simulink model "baseline_auto_parcel_loading_process"  (R2026a)
settings: Solver=VariableStepAuto  StopTime=500  MaxStep=0.05
libraries: sim3dlib x36
(part 2 of 5)

== matlab function baseline_auto_parcel_loading_process/BoxSizeFunction ==
  data: box_type output; box_length output; box_width output; box_height output; load_done input; package_count output
function [box_type, box_length, box_width, box_height, package_count] = BoxSizeFunction(load_done)
% BoxSizeFunction
% 연속 상차용 랜덤 택배 크기 생성 함수
%
% load_done이 0 -> 1로 바뀌는 순간,
% 다음 상차 사이클에서 사용할 새 택배 종류를 랜덤 생성한다.
%
% 출력 단위:
% box_length, box_width, box_height = m

persistent selected_type
persistent count
persistent prev_load_done

if isempty(selected_type)
    selected_type = randi(4);
    count = 1;
    prev_load_done = 0;
end

% load_done 상승 에지 감지
rising_edge = (prev_load_done == 0) && (load_done == 1);

% 상차 완료 순간 다음 택배 생성
if rising_edge
    selected_type = randi(4);
    count = count + 1;
end

prev_load_done = load_done;

box_type = selected_type;
package_count = count;

% 우체국 택배 1~4호 예시 치수
% 실제 제작 박스 치수에 맞춰 나중에 수정 가능
% [length, width, height], 단위: m
if box_type == 1
    real_length = 0.220;
    real_width  = 0.190;
    real_height = 0.090;
elseif box_type == 2
    real_length = 0.270;
    real_width  = 0.180;
    real_height = 0.150;
elseif box_type == 3
    real_length = 0.340;
    real_width  = 0.250;
    real_height = 0.210;
else
    real_length = 0.410;
    real_width  = 0.310;
    real_height = 0.280;
end

% 2:1 축소 스케일
scale = 0.5;

box_length = real_length * scale;
box_width  = real_width  * scale;
box_height = real_height * scale;

== stateflow chart baseline_auto_parcel_loading_process/MainController ==
  state LOAD_FINISHED
    entry:
    lift_cmd = 0;
    target_z = 0.0;
    state_id = 14;
    door_cmd = 0;
    platform_fold_cmd = 0;
    rotator_cmd = 0;
    pusher_cmd = 0;
    % 핵심: 상차 phase 종료이므로 스토퍼 올림
    stopper_cmd = 0;
    floor1_conv_cmd = 0;
    floor2_conv_cmd = 0;
    floor3_conv_cmd = 0;
    load_done = 0;
    spawn_pkg = 0;
  state NO_STORAGE
    entry:
    lift_cmd = 0;
    target_z = 0.0;
    state_id = 13;
    door_cmd = 1;
    platform_fold_cmd = 1;
    rotator_cmd = 0;
    pusher_cmd = 0;
    stopper_cmd = 0;
    floor1_conv_cmd = 0;
    floor2_conv_cmd = 0;
    floor3_conv_cmd = 0;
    load_done = 0;
    spawn_pkg = 0;
  state ROTATOR_RETURN_HOME
    entry:
    lift_cmd = 0;
    target_z = 0.0;
    state_id = 15;
    door_cmd = 1;
    platform_fold_cmd = 1;
    rotator_cmd = 2;
    pusher_cmd = 0;
    stopper_cmd = 0;
    floor1_conv_cmd = 0;
    floor2_conv_cmd = 0;
    floor3_conv_cmd = 0;
    load_done = 0;
    spawn_pkg = 0;
  state COMPLETE
    entry:
    lift_cmd = 0;
    target_z = 0.0;
    state_id = 12;
    door_cmd = 1;
    platform_fold_cmd = 1;
    rotator_cmd = 0;
    pusher_cmd = 0;
    stopper_cmd = 0;
    floor1_conv_cmd = 0;
    floor2_conv_cmd = 0;
    floor3_conv_cmd = 0;
    load_done = 0;
    spawn_pkg = 0;
  state IDLE
    entry:
    lift_cmd = 0;
    target_z = 0.0;
    state_id = 0;
    door_cmd = 1;
    platform_fold_cmd = 1;
    rotator_cmd = 0;
    pusher_cmd = 0;
    stopper_cmd = 0;
    floor1_conv_cmd = 0;
    floor2_conv_cmd = 0;
    floor3_conv_cmd = 0;
    load_done = 0;
    spawn_pkg = 0;
  state SELECT_TARGET_FLOOR
    entry:
    lift_cmd = 0;
    if target_floor == 1
    target_z = 0.0;
    elseif target_floor == 2
    target_z = 0.27;
    elseif target_floor == 3
    target_z = 0.54;
    else
    target_z = 0.0;
    end
    state_id = 4;
    door_cmd = 1;
    platform_fold_cmd = 1;
    rotator_cmd = 0;
    pusher_cmd = 0;
    stopper_cmd = 0;
    floor1_conv_cmd = 0;
    floor2_conv_cmd = 0;
    floor3_conv_cmd = 0;
    load_done = 0;
    spawn_pkg = 0;
  state WAIT_PACKAGE
    entry:
    lift_cmd = 0;
    target_z = 0.0;
    state_id = 2;
    door_cmd = 1;
    platform_fold_cmd = 1;
    rotator_cmd = 0;
    pusher_cmd = 0;
    stopper_cmd = 0;
    floor1_conv_cmd = 0;
    floor2_conv_cmd = 0;
    floor3_conv_cmd = 0;
    load_done = 0;
    spawn_pkg = 1;
  state SCAN_AND_ROTATE
    entry:
    lift_cmd = 0;
    target_z = 0.0;
    state_id = 3;
    door_cmd = 1;
    platform_fold_cmd = 1;
    rotator_cmd = 1;
    pusher_cmd = 0;
    stopper_cmd = 0;
    floor1_conv_cmd = 0;
    floor2_conv_cmd = 0;
    floor3_conv_cmd = 0;
    load_done = 0;
    spawn_pkg = 0;
  state MOVE_TO_TARGET_FLOOR
    during:
    if target_floor == 1
    target_z = 0.0;
    elseif target_floor == 2
    target_z = 0.27;
    elseif target_floor == 3
    target_z = 0.54;
    else
    target_z = 0.0;
    end
    if platform_z < target_z - 0.0001
    lift_cmd = 1;
    else
    lift_cmd = 0;
    end
    state_id = 5;
    door_cmd = 1;
    platform_fold_cmd = 1;
    rotator_cmd = 0;
    pusher_cmd = 0;
    stopper_cmd = 0;
    floor1_conv_cmd = 0;
    floor2_conv_cmd = 0;
    floor3_conv_cmd = 0;
    load_done = 0;
    spawn_pkg = 0;
  state PLATFORM_UNFOLD
    entry:
    lift_cmd = 0;
    target_z = 0.0;
    state_id = 1;
    door_cmd = 1;
    platform_fold_cmd = 1;
    rotator_cmd = 0;
    pusher_cmd = 0;
    stopper_cmd = 0;
    floor1_conv_cmd = 0;
    floor2_conv_cmd = 0;
    floor3_conv_cmd = 0;
    load_done = 0;
    spawn_pkg = 0;
  state LOAD_REGISTER
    entry:
    lift_cmd = 0;
    if target_floor == 1
    target_z = 0.0;
    floor1_conv_cmd = 0;
    floor2_conv_cmd = 0;
    floor3_conv_cmd = 0;
    elseif target_floor == 2
    target_z = 0.27;
    floor1_conv_cmd = 0;
    floor2_conv_cmd = 0;
    floor3_conv_cmd = 0;
    elseif target_floor == 3
    target_z = 0.54;
    floor1_conv_cmd = 0;
    floor2_conv_cmd = 0;
    floor3_conv_cmd = 0;
    else
    target_z = 0.0;
    floor1_conv_cmd = 0;
    floor2_conv_cmd = 0;
    floor3_conv_cmd = 0;
    end
    state_id = 17;
    door_cmd = 1;
    platform_fold_cmd = 1;
    rotator_cmd = 0;
    pusher_cmd = 0;
    % 핵심: 아직 상차 phase 중이므로 스토퍼는 계속 내려둔다
    stopper_cmd = 1;
    % 여기서 상차 완료 신호 발생
    load_done = 1;
    spawn_pkg = 0;
  state PUSH_TO_BELT4
    entry:
    lift_cmd = 0;
    if target_floor == 1
    target_z = 0.0;
    floor1_conv_cmd = 1;
    floor2_conv_cmd = 0;
    floor3_conv_cmd = 0;
    elseif target_floor == 2
    target_z = 0.27;
    floor1_conv_cmd = 0;
    floor2_conv_cmd = 1;
    floor3_conv_cmd = 0;
    elseif target_floor == 3
    target_z = 0.54;
    floor1_conv_cmd = 0;
    floor2_conv_cmd = 0;
    floor3_conv_cmd = 1;
    else
    target_z = 0.0;
    floor1_conv_cmd = 0;
    floor2_conv_cmd = 0;
    floor3_conv_cmd = 0;
    end
    state_id = 7;
    door_cmd = 1;
    platform_fold_cmd = 1;
    rotator_cmd = 0;
    pusher_cmd = 1;
    stopper_cmd = 1;
    load_done = 0;
    spawn_pkg = 0;
  state PACKING
    entry:
    lift_cmd = 0;
    if target_floor == 1
    target_z = 0.0;
    floor1_conv_cmd = 1;
    floor2_conv_cmd = 0;
    floor3_conv_cmd = 0;
    elseif target_floor == 2
    target_z = 0.27;
    floor1_conv_cmd = 0;
    floor2_conv_cmd = 1;
    floor3_conv_cmd = 0;
    elseif target_floor == 3
    target_z = 0.54;
    floor1_conv_cmd = 0;
    floor2_conv_cmd = 0;
    floor3_conv_cmd = 1;
    else
    target_z = 0.0;
    floor1_conv_cmd = 1;
    floor2_conv_cmd = 0;
    floor3_conv_cmd = 0;
    end
    state_id = 8;
    door_cmd = 1;
    platform_fold_cmd = 1;
    rotator_cmd = 0;
    pusher_cmd = 0;
    stopper_cmd = 1;
    load_done = 0;
    spawn_pkg = 0;
  state PUSHER_RETURN_HOME
    entry:
    lift_cmd = 0;
    if target_floor == 1
    target_z = 0.0;
    floor1_conv_cmd = 1;
    floor2_conv_cmd = 0;
    floor3_conv_cmd = 0;
    elseif target_floor == 2
    target_z = 0.27;
    floor1_conv_cmd = 0;
    floor2_conv_cmd = 1;
    floor3_conv_cmd = 0;
    elseif target_floor == 3
    target_z = 0.54;
    floor1_conv_cmd = 0;
    floor2_conv_cmd = 0;
    floor3_conv_cmd = 1;
    else
    target_z = 0.0;
    floor1_conv_cmd = 0;
    floor2_conv_cmd = 0;
    floor3_conv_cmd = 0;
    end
    state_id = 16;
    door_cmd = 1;
    platform_fold_cmd = 1;
    rotator_cmd = 0;
    pusher_cmd = 2;
    stopper_cmd = 1;
    load_done = 0;
    spawn_pkg = 0;
  state MOVE_DOWN
    entry:
    target_z = 0.0;
    lift_cmd = -1;
    state_id = 10;
    door_cmd = 1;
    platform_fold_cmd = 1;
    rotator_cmd = 0;
    pusher_cmd = 0;
    stopper_cmd = 1;
    floor1_conv_cmd = 0;
    floor2_conv_cmd = 0;
    floor3_conv_cmd = 0;
    spawn_pkg = 0;
  state PLATFORM_FOLD
    entry:
    lift_cmd = 0;
    target_z = 0.0;
    state_id = 11;
    door_cmd = 1;
    platform_fold_cmd = 0;
    rotator_cmd = 0;
    pusher_cmd = 0;
    stopper_cmd = 0;
    floor1_conv_cmd = 0;
    floor2_conv_cmd = 0;
    floor3_conv_cmd = 0;
    spawn_pkg = 0;
  state STOPPER_DOWN
    entry:
    lift_cmd = 0;
    if target_floor == 1
    target_z = 0.0;
    elseif target_floor == 2
    target_z = 0.27;
    elseif target_floor == 3
    target_z = 0.54;
    else
    target_z = 0.0;
    end
    state_id = 6;
    door_cmd = 1;
    platform_fold_cmd = 1;
    rotator_cmd = 0;
    pusher_cmd = 0;
    stopper_cmd = 1;
    floor1_conv_cmd = 0;
    floor2_conv_cmd = 0;
    floor3_conv_cmd = 0;
    load_done = 0;
    spawn_pkg = 0;
  IDLE -> LOAD_FINISHED [order 2] : [after(1, sec) && loading_enable == 0]
  COMPLETE -> LOAD_FINISHED [order 2] : [after(1, sec) && loading_enable == 0]
  SELECT_TARGET_FLOOR -> NO_STORAGE [order 2] : [storage_available == 0]
  (default) -> IDLE
  IDLE -> PLATFORM_UNFOLD [order 1] : [after(1, sec) && loading_enable == 1]
  SELECT_TARGET_FLOOR -> MOVE_TO_TARGET_FLOOR [order 1] : [storage_available == 1]
  COMPLETE -> IDLE [order 1] : [after(1, sec) && loading_enable == 1]
  SCAN_AND_ROTATE -> ROTATOR_RETURN_HOME : [rotation_done == 1]
  ROTATOR_RETURN_HOME -> SELECT_TARGET_FLOOR : [rotator_home_done == 1]
  PLATFORM_UNFOLD -> WAIT_PACKAGE : [after(1, sec)]
  WAIT_PACKAGE -> SCAN_AND_ROTATE : [after(1, sec)]
  PLATFORM_FOLD -> COMPLETE : [after(1, sec)]
  MOVE_TO_TARGET_FLOOR -> STOPPER_DOWN : [platform_z >= target_z - 0.0001]
  MOVE_DOWN -> PLATFORM_FOLD : [platform_z <= 0.0001]
  LOAD_REGISTER -> MOVE_DOWN : [after(0.1, sec)]
  STOPPER_DOWN -> PUSH_TO_BELT4 : [stopper_down_done == 1]
  PACKING -> LOAD_REGISTER : [moving_arrive_done == 1]
  PUSHER_RETURN_HOME -> PACKING : [pusher_home_done == 1]
  PUSH_TO_BELT4 -> PUSHER_RETURN_HOME : [push_done == 1]
  data: target_floor input; platform_z input; lift_cmd output; target_z output; state_id output; door_cmd output; platform_fold_cmd output; rotator_cmd output; pusher_cmd output; stopper_cmd output; floor1_conv_cmd output; floor2_conv_cmd output; floor3_conv_cmd output; load_done output; storage_available input; loading_enable input; rotation_done input; rotator_home_done input; push_done input; pusher_home_done input; stopper_down_done input; spawn_pkg output; moving_arrive_done input

== matlab function baseline_auto_parcel_loading_process/BoxRotationFunction ==
  data: box_length input; box_insert_length output; box_width input; desired_box_yaw output; box_yaw input; rotator_target_angle output
function [box_insert_length, desired_box_yaw, rotator_target_angle] = BoxRotationFunction(box_length, box_width, box_yaw)
% BoxRotationFunction
% 랜덤하게 놓인 택배 yaw를 기준으로,
% 컨베이어 진행방향 점유 길이가 최소가 되도록 필요한 회전각을 계산한다.
%
% 입력:
%   box_length : 택배 긴 방향 길이 [m]
%   box_width  : 택배 짧은 방향 길이 [m]
%   box_yaw    : 카메라/YOLO가 인식한 현재 택배 yaw [deg]
%
% 출력:
%   box_insert_length     : 회전 후 컨베이어 진행방향으로 차지하는 길이 [m]
%   desired_box_yaw       : 목표 택배 yaw [deg]
%   rotator_target_angle  : 회전판이 회전해야 하는 보정각 [deg]

% 적재 효율을 위해 짧은 변이 진행방향을 향하도록 한다.
% 여기서는 단순히:
% - box_length <= box_width이면 현재 0 deg 방향이 유리
% - box_length > box_width이면 90 deg 방향이 유리
%
% 실제로는 카메라 좌표계와 컨베이어 진행방향 정의에 따라
% desired_box_yaw 기준을 조정해야 한다.

if box_length <= box_width
    box_insert_length = box_length;
    desired_box_yaw = 0;
else
    box_insert_length = box_width;
    desired_box_yaw = 90;
end

% 현재 yaw에서 목표 yaw까지 필요한 회전각
raw_angle = desired_box_yaw - box_yaw;

% 회전각을 -90 ~ 90 deg 범위로 정규화
rotator_target_angle = normalizeToMinus90To90(raw_angle);


function angle_out = normalizeToMinus90To90(angle_in)
% angle_in을 -90 ~ 90 범위로 정규화

angle_out = angle_in;

while angle_out > 90
    angle_out = angle_out - 180;
end

while angle_out < -90
    angle_out = angle_out + 180;
end

== matlab function baseline_auto_parcel_loading_process/FloorStorageUpdate ==
  data: load_done input; floor1_used_length output; target_floor input; box_insert_length input; floor2_used_length output; floor3_used_length output; floor1_count output; floor2_count output; floor3_count output; package_id input; floor1_queue output; floor2_queue output; floor3_queue output; unload_done input; target_package_id input; target_unload_floor input; target_package_length output
function [floor1_used_length, floor2_used_length, floor3_used_length, floor1_count, floor2_count, floor3_count, floor1_queue, floor2_queue, floor3_queue, target_package_length] = FloorStorageUpdate(load_done, target_floor, box_insert_length, package_id, unload_done, target_package_id, target_unload_floor)
% FloorStorageUpdate
% 상차 완료 시:
%   1) 선택된 층 used_length 증가
%   2) 선택된 층 count 증가
%   3) 선택된 층 queue 뒤에 package_id 저장
%   4) package_id별 box_insert_length 저장
%
% 하차 완료 시:
%   1) 대상 층 queue에서 target_package_id 삭제
%   2) 대상 층 count 감소
%   3) target_package_id에 저장된 길이만큼 used_length 감소
%
% queue는 column vector [QUEUE_MAX x 1] 형태로 통일한다.

persistent f1_used f2_used f3_used
persistent f1_count f2_count f3_count
persistent q1 q2 q3
persistent package_lengths
persistent prev_load_done prev_unload_done

QUEUE_MAX = 50;
PACKAGE_MAX = 1000;

if isempty(f1_used)
    % 초기 적재 길이
    f1_used = 0.40;
    f2_used = 0.45;
    f3_used = 0.20;

    % 이번 시뮬레이션에서 새로 상차된 택배 개수
    f1_count = 0;
    f2_count = 0;
    f3_count = 0;

    % 층별 큐: column vector로 통일
    q1 = zeros(QUEUE_MAX, 1);
    q2 = zeros(QUEUE_MAX, 1);
    q3 = zeros(QUEUE_MAX, 1);

    % package_id별 택배 진행방향 길이 저장
    package_lengths = zeros(PACKAGE_MAX, 1);

    prev_load_done = 0;
    prev_unload_done = 0;
end

% 상승 에지 감지
load_rising_edge = (prev_load_done == 0) && (load_done == 1);
unload_rising_edge = (prev_unload_done == 0) && (unload_done == 1);

% 현재 target_package_id의 저장된 길이 조회
target_idx = int32(target_package_id);
target_package_length = 0;

if target_idx >= 1 && target_idx <= PACKAGE_MAX
    target_package_length = package_lengths(target_idx);
end

% =========================
% 상차 업데이트
% =========================
if load_rising_edge
    pkg_idx = int32(package_id);

    % package_id별 길이 저장
    if pkg_idx >= 1 && pkg_idx <= PACKAGE_MAX
        package_lengths(pkg_idx) = box_insert_length;
    end

    if target_floor == 1
        if f1_count < QUEUE_MAX
            f1_count = f1_count + 1;
            q1(f1_count) = package_id;
            f1_used = f1_used + box_insert_length;
        end

    elseif target_floor == 2
        if f2_count < QUEUE_MAX
            f2_count = f2_count + 1;
            q2(f2_count) = package_id;
            f2_used = f2_used + box_insert_length;
        end

    elseif target_floor == 3
        if f3_count < QUEUE_MAX
            f3_count = f3_count + 1;
            q3(f3_count) = package_id;
            f3_used = f3_used + box_insert_length;
        end
    end
end

% =========================
% 하차 업데이트
% =========================
if unload_rising_edge
    target_idx_for_unload = int32(target_package_id);
    removed_length = 0;

    if target_idx_for_unload >= 1 && target_idx_for_unload <= PACKAGE_MAX
        removed_length = package_lengths(target_idx_for_unload);
    end

    % 혹시 길이가 저장되어 있지 않으면 안전하게 현재 box_insert_length 사용
    if removed_length <= 0
        removed_length = box_insert_length;
    end

    if target_unload_floor == 1
        [q1, f1_count, removed] = removePackageFromQueue(q1, f1_count, target_package_id, QUEUE_MAX);

        if removed == 1
            f1_used = f1_used - removed_length;

            if f1_used < 0
                f1_used = 0;
            end

            if target_idx_for_unload >= 1 && target_idx_for_unload <= PACKAGE_MAX
                package_lengths(target_idx_for_unload) = 0;
            end
        end

    elseif target_unload_floor == 2
        [q2, f2_count, removed] = removePackageFromQueue(q2, f2_count, target_package_id, QUEUE_MAX);

        if removed == 1
            f2_used = f2_used - removed_length;

            if f2_used < 0
                f2_used = 0;
            end

            if target_idx_for_unload >= 1 && target_idx_for_unload <= PACKAGE_MAX
                package_lengths(target_idx_for_unload) = 0;
            end
        end

    elseif target_unload_floor == 3
        [q3, f3_count, removed] = removePackageFromQueue(q3, f3_count, target_package_id, QUEUE_MAX);

        if removed == 1
            f3_used = f3_used - removed_length;

            if f3_used < 0
                f3_used = 0;
            end

            if target_idx_for_unload >= 1 && target_idx_for_unload <= PACKAGE_MAX
                package_lengths(target_idx_for_unload) = 0;
            end
        end
    end
end

prev_load_done = load_done;
prev_unload_done = unload_done;

% 하차 업데이트 이후 target_package_length 다시 계산
target_idx = int32(target_package_id);
target_package_length = 0;

if target_idx >= 1 && target_idx <= PACKAGE_MAX
    target_package_length = package_lengths(target_idx);
end

floor1_used_length = f1_used;
floor2_used_length = f2_used;
floor3_used_length = f3_used;

floor1_count = f1_count;
floor2_count = f2_count;
floor3_count = f3_count;

floor1_queue = q1;
floor2_queue = q2;
floor3_queue = q3;


function [q_out, count_out, removed] = removePackageFromQueue(q_in, count_in, target_id, queue_max)
% q_in에서 target_id를 찾아 삭제하고, 뒤쪽 원소들을 앞으로 당긴다.

q_out = q_in;
count_out = count_in;
removed = 0;

remove_idx = 0;

for i = 1:queue_max
    if q_out(i) == target_id
        remove_idx = i;
        removed = 1;
        break;
    end
end

if removed == 1
    % 삭제 위치부터 한 칸씩 앞으로 당김
    for i = remove_idx:(queue_max - 1)
        q_out(i) = q_out(i + 1);
    end

    % 마지막 칸 비우기
    q_out(queue_max) = 0;

    % count 감소
    if count_out > 0
        count_out = count_out - 1;
    end
end

== matlab function baseline_auto_parcel_loading_process/TargetPackageFinder ==
  data: target_package_id input; target_found output; floor1_queue input; floor2_queue input; floor3_queue input; target_unload_floor output; target_package_index output
function [target_found, target_unload_floor, target_package_index] = TargetPackageFinder(target_package_id, floor1_queue, floor2_queue, floor3_queue)
% TargetPackageFinder
% target_package_id가 각 층 queue 중 어디에 있는지 찾는다.
%
% target_found:
%   0 = 못 찾음
%   1 = 찾음
%
% target_unload_floor:
%   0 = 못 찾음
%   1 = 1층
%   2 = 2층
%   3 = 3층
%
% target_package_index:
%   해당 층 queue 안에서 몇 번째인지
%   예: floor2_queue = [1 2 4 0 ...]에서 target_package_id=4이면 index=3

target_found = 0;
target_unload_floor = 0;
target_package_index = 0;

QUEUE_MAX = 50;

% 1층 검색
for i = 1:QUEUE_MAX
    if floor1_queue(i) == target_package_id
        target_found = 1;
        target_unload_floor = 1;
        target_package_index = i;
        return;
    end
end

% 2층 검색
for i = 1:QUEUE_MAX
    if floor2_queue(i) == target_package_id
        target_found = 1;
        target_unload_floor = 2;
        target_package_index = i;
        return;
    end
end

% 3층 검색
for i = 1:QUEUE_MAX
    if floor3_queue(i) == target_package_id
        target_found = 1;
        target_unload_floor = 3;
        target_package_index = i;
        return;
    end
end

== matlab function baseline_auto_parcel_loading_process/UnloadPrepositionFunction ==
  data: unload_request input; preposition_active output; vehicle_stopped input; target_found input; target_unload_floor input; target_package_index input; sensor_count output; target_package_on_belt4 output; unload_floor1_conv_cmd output; unload_floor2_conv_cmd output; unload_floor3_conv_cmd output
function [preposition_active, sensor_count, target_package_on_belt4, unload_floor1_conv_cmd, unload_floor2_conv_cmd, unload_floor3_conv_cmd] = UnloadPrepositionFunction(unload_request, vehicle_stopped, target_found, target_unload_floor, target_package_index)
% UnloadPrepositionFunction
%
% 배송 중 하차 준비 단계 모델
%
% 목적:
% - 상차 완료 후 unload_request가 1이 되면 하차 준비 가능 상태가 된다.
% - 차량이 정차 중(vehicle_stopped == 1)일 때만 대상 층 컨베이어를 순환시킨다.
% - 모든 택배는 순서를 유지한 채 함께 순환한다고 가정한다.
% - target_package_index 위치의 택배가 slot 1, 즉 Belt4 상단/플랫폼 앞 하차공간에 오면
%   target_package_on_belt4 = 1 로 만든다.
%
% 핵심:
% - target_package_index = 1이면 이미 하차공간에 있는 것으로 판단한다.
% - target_package_index = 4이면 3칸 순환하면 하차공간에 온다.
%
% 출력:
% preposition_active       : 하차 준비 순환 중이면 1
% sensor_count             : 현재까지 순환된 칸 수
% target_package_on_belt4  : 대상 택배가 하차공간에 준비되면 1
% unload_floorN_conv_cmd   : 대상 층 순환 컨베이어 구동 명령

persistent count
persistent active
persistent done
persistent step_counter
persistent prev_unload_request
persistent last_target_floor
persistent last_target_index

% 몇 계산 step마다 택배 1개가 센서/하차공간 기준으로 이동했다고 볼지
% 값이 작을수록 순환 준비가 빠르게 보임
COUNT_INTERVAL = 20;

if isempty(count)
    count = 0;
    active = 0;
    done = 0;
    step_counter = 0;
    prev_unload_request = 0;
    last_target_floor = 0;
    last_target_index = 0;
end

% 기본 출력
preposition_active = active;
sensor_count = count;
target_package_on_belt4 = done;

unload_floor1_conv_cmd = 0;
unload_floor2_conv_cmd = 0;
unload_floor3_conv_cmd = 0;

% 하차 요청 상승 에지 감지
request_rising = (prev_unload_request == 0) && (unload_request == 1);

% 대상이 바뀌었는지도 확인
target_changed = (target_unload_floor ~= last_target_floor) || ...
                 (target_package_index ~= last_target_index);

% 새 하차 요청이 들어오거나 대상이 바뀌면 초기화
if request_rising || target_changed
    count = 0;
    active = 0;
    done = 0;
    step_counter = 0;

    last_target_floor = target_unload_floor;
    last_target_index = target_package_index;
end

prev_unload_request = unload_request;

% 유효하지 않은 조건이면 정지
if unload_request < 0.5 || target_found < 0.5 || target_unload_floor < 1 || target_unload_floor > 3 || target_package_index < 1
    active = 0;
    done = 0;
    count = 0;
    step_counter = 0;

    preposition_active = active;
    sensor_count = count;
    target_package_on_belt4 = done;
    return;
end

% target_package_index가 1이면 이미 Belt4 상단/플랫폼 앞 하차공간에 있다고 본다.
required_shift = target_package_index - 1;

if required_shift < 0
    required_shift = 0;
end

% 이미 필요한 만큼 순환했으면 준비 완료
if count >= required_shift
    active = 0;
    done = 1;

    unload_floor1_conv_cmd = 0;
    unload_floor2_conv_cmd = 0;
    unload_floor3_conv_cmd = 0;

    preposition_active = active;
    sensor_count = count;
    target_package_on_belt4 = done;
    return;
end

% 아직 준비가 안 끝났고, 차량이 정차 중이면 순환 시작/유지
if vehicle_stopped > 0.5
    active = 1;
else
    % 배송 중이지만 정차 상태가 아니면 현재 위치에서 멈춤
    active = 0;
end

% 하차 준비 동작
if active == 1 && done == 0

    % 대상 층 컨베이어만 순환
    if target_unload_floor == 1
        unload_floor1_conv_cmd = 1;
        unload_floor2_conv_cmd = 0;
        unload_floor3_conv_cmd = 0;

    elseif target_unload_floor == 2
        unload_floor1_conv_cmd = 0;
        unload_floor2_conv_cmd = 1;
        unload_floor3_conv_cmd = 0;

    elseif target_unload_floor == 3
        unload_floor1_conv_cmd = 0;
        unload_floor2_conv_cmd = 0;
        unload_floor3_conv_cmd = 1;
    end

    % 가상 센서/순환 카운트
    step_counter = step_counter + 1;

    if step_counter >= COUNT_INTERVAL
        step_counter = 0;
        count = count + 1;
    end

    % 필요한 순환 수에 도달하면 준비 완료
    if count >= required_shift
        done = 1;
        active = 0;

        unload_floor1_conv_cmd = 0;
        unload_floor2_conv_cmd = 0;
        unload_floor3_conv_cmd = 0;
    end
end

preposition_active = active;
sensor_count = count;
target_package_on_belt4 = done;

end

== stateflow chart baseline_auto_parcel_loading_process/UnloadController ==
  state U_IDLE
    during:
    unload_state_id = 0;
    belt4_reverse_cmd = 0;
    belt4_restore_cmd = 0;
    package_on_platform_from_floor = 0;
    unload_done = 0;
    % 기본 목표는 1층 복귀
    unload_target_z = 0.00;
    % 배송 중 하차 준비 단계에서는 실제 하차 전이므로
    % 플랫폼을 항상 1층으로 복귀시킨다.
    if delivery_arrived < 0.5
    if platform_z > 0.005
    unload_lift_cmd = -1;
    elseif platform_z < -0.005
    unload_lift_cmd = 1;
    else
    unload_lift_cmd = 0;
    end
    else
    % 배달 장소 도착 후에는 다음 하차 상태 전이를 기다림
    unload_lift_cmd = 0;
    end
  state U_WAIT_READY
    entry:
    unload_lift_cmd = 0;
    unload_target_z = 0.0;
    unload_state_id = 1;
    belt4_reverse_cmd = 0;
    belt4_restore_cmd = 0;
    package_on_platform_from_floor = 0;
    unload_done = 0;
  state U_MOVE_TO_TARGET_FLOOR
    during:
    unload_state_id = 2;
    belt4_reverse_cmd = 0;
    belt4_restore_cmd = 0;
    package_on_platform_from_floor = 0;
    unload_done = 0;
    if target_unload_floor == 1
    unload_target_z = 0.00;
    elseif target_unload_floor == 2
    unload_target_z = 0.27;
    elseif target_unload_floor == 3
    unload_target_z = 0.54;
    else
    unload_target_z = 0.00;
    end
    if platform_z < unload_target_z - 0.005
    unload_lift_cmd = 1;
    elseif platform_z > unload_target_z + 0.005
    unload_lift_cmd = -1;
    else
    unload_lift_cmd = 0;
    end
  state U_REVERSE_BELT4
    entry:
    unload_lift_cmd = 0;
    if target_unload_floor == 1
    unload_target_z = 0.0;
    elseif target_unload_floor == 2
    unload_target_z = 0.27;
    elseif target_unload_floor == 3
    unload_target_z = 0.54;
    else
    unload_target_z = 0.0;
    end
    unload_state_id = 3;
    belt4_reverse_cmd = 1;
    belt4_restore_cmd = 0;
    package_on_platform_from_floor = 0;
    unload_done = 0;
  state U_PACKAGE_ON_PLATFORM
    entry:
    unload_lift_cmd = 0;
    if target_unload_floor == 1
    unload_target_z = 0.0;
    elseif target_unload_floor == 2
    unload_target_z = 0.27;
    elseif target_unload_floor == 3
    unload_target_z = 0.54;
    else
    unload_target_z = 0.0;
    end
    unload_state_id = 4;
    belt4_reverse_cmd = 0;
    belt4_restore_cmd = 0;
    package_on_platform_from_floor = 1;
    unload_done = 0;
  state U_COMPLETE
    entry:
    unload_lift_cmd = 0;
    unload_target_z = 0.0;
    unload_state_id = 7;
    belt4_reverse_cmd = 0;
    belt4_restore_cmd = 0;
    package_on_platform_from_floor = 1;
    unload_done = 1;
  state U_RESTORE_BELT4
    entry:
    unload_lift_cmd = 0;
    if target_unload_floor == 1
    unload_target_z = 0.0;
    elseif target_unload_floor == 2
    unload_target_z = 0.27;
    elseif target_unload_floor == 3
    unload_target_z = 0.54;
    else
    unload_target_z = 0.0;
    end
    unload_state_id = 5;
    belt4_reverse_cmd = 0;
    belt4_restore_cmd = 1;
    package_on_platform_from_floor = 1;
    unload_done = 0;
  state U_MOVE_DOWN
    during:
    unload_target_z = 0.0;
    if platform_z > 0.0001
    unload_lift_cmd = -1;
    else
    unload_lift_cmd = 0;
    end
    unload_state_id = 6;
    belt4_reverse_cmd = 0;
    belt4_restore_cmd = 0;
    package_on_platform_from_floor = 1;
    unload_done = 0;
  (default) -> U_IDLE
  U_WAIT_READY -> U_MOVE_TO_TARGET_FLOOR : [delivery_arrived == 1]
  U_MOVE_TO_TARGET_FLOOR -> U_REVERSE_BELT4 : [(target_unload_floor == 1 && platform_z >= -0.005 && platform_z <= 0.005) || ...
      |  (target_unload_floor == 2 && platform_z >= 0.265 && platform_z <= 0.275) || ...
      |  (target_unload_floor == 3 && platform_z >= 0.535 && platform_z <= 0.545)]
  U_REVERSE_BELT4 -> U_PACKAGE_ON_PLATFORM : [after(1.5, sec)]
  U_IDLE -> U_WAIT_READY : [delivery_arrived > 0.5 && platform_deployed > 0.5 && target_package_on_belt4 > 0.5]
  U_COMPLETE -> U_IDLE : [after(0.1, sec)]
  U_PACKAGE_ON_PLATFORM -> U_RESTORE_BELT4 : [after(0.5, sec)]
  U_MOVE_DOWN -> U_COMPLETE : [platform_z <= 0.0001]
  U_RESTORE_BELT4 -> U_MOVE_DOWN : [after(1.5, sec)]
  data: target_package_on_belt4 input; target_unload_floor input; platform_z input; delivery_arrived input; unload_lift_cmd output; unload_target_z output; unload_state_id output; belt4_reverse_cmd output; belt4_restore_cmd output; package_on_platform_from_floor output; unload_done output; platform_deployed input

== matlab function baseline_auto_parcel_loading_process/MissionModeFunction ==
  data: floor1_count input; loading_enable output; floor2_count input; floor3_count input; load_target_count input; unload_request_auto output; total_loaded_count output; unload_done input; mission_phase output
function [loading_enable, unload_request_auto, total_loaded_count, mission_phase] = MissionModeFunction(floor1_count, floor2_count, floor3_count, load_target_count, unload_done)
% MissionModeFunction
%
% mission_phase:
% 0 = 상차 단계
% 1 = 하차 준비/하차 단계
% 2 = 전체 미션 완료

persistent phase
persistent prev_unload_done

if isempty(phase)
    phase = 0;
    prev_unload_done = 0;
end

total_loaded_count = floor1_count + floor2_count + floor3_count;

unload_rising_edge = (prev_unload_done == 0) && (unload_done == 1);

% 상차 완료 → 하차 단계
if phase == 0
    if total_loaded_count >= load_target_count
        phase = 1;
    end
end

% 모든 하차 대상 완료 → 미션 완료
if phase == 1
    if unload_rising_edge
        phase = 2;
    end
end

prev_unload_done = unload_done;

if phase == 0
    loading_enable = 1;
    unload_request_auto = 0;

elseif phase == 1
    loading_enable = 0;
    unload_request_auto = 1;

else
    loading_enable = 0;
    unload_request_auto = 0;
end

mission_phase = phase;

end

== matlab function baseline_auto_parcel_loading_process/CommandMuxFunction ==
  data: mission_phase input; final_lift_cmd output; load_lift_cmd input; load_target_z input; load_floor1_conv_cmd input; load_floor2_conv_cmd input; load_floor3_conv_cmd input; pre_floor1_conv_cmd input; pre_floor2_conv_cmd input; pre_floor3_conv_cmd input; unload_lift_cmd input; unload_target_z input; target_unload_floor input; belt4_reverse_cmd input; belt4_restore_cmd input; final_target_z output; final_floor1_conv_cmd output; final_floor2_conv_cmd output; final_floor3_conv_cmd output; final_floor1_belt4_cmd output; final_floor2_belt4_cmd output; final_floor3_belt4_cmd output
function [final_lift_cmd, final_target_z, ...
          final_floor1_conv_cmd, final_floor2_conv_cmd, final_floor3_conv_cmd, ...
          final_floor1_belt4_cmd, final_floor2_belt4_cmd, final_floor3_belt4_cmd] = ...
          CommandMuxFunction(mission_phase, ...
          load_lift_cmd, load_target_z, load_floor1_conv_cmd, load_floor2_conv_cmd, load_floor3_conv_cmd, ...
          pre_floor1_conv_cmd, pre_floor2_conv_cmd, pre_floor3_conv_cmd, ...
          unload_lift_cmd, unload_target_z, target_unload_floor, belt4_reverse_cmd, belt4_restore_cmd)
% CommandMuxFunction
% mission_phase에 따라 상차/하차 명령을 최종 장치 명령으로 선택한다.
%
% mission_phase:
%   0 = 상차 단계
%   1 = 하차 단계
%   2 = 미션 완료
%
% final_floorN_conv_cmd:
%   1 = 해당 층 전체 순환 컨베이어 시계방향 회전
%   0 = 정지
%
% final_floorN_belt4_cmd:
%  -1 = 4번 벨트 역회전, 택배를 플랫폼으로 하차
%   0 = 정지
%   1 = 4번 벨트 정방향 복귀

% 기본값: 전체 정지
final_lift_cmd = 0;
final_target_z = 0.0;

final_floor1_conv_cmd = 0;
final_floor2_conv_cmd = 0;
final_floor3_conv_cmd = 0;

final_floor1_belt4_cmd = 0;
final_floor2_belt4_cmd = 0;
final_floor3_belt4_cmd = 0;

% =========================
% 상차 단계
% =========================
if mission_phase == 0
    final_lift_cmd = load_lift_cmd;
    final_target_z = load_target_z;

    final_floor1_conv_cmd = load_floor1_conv_cmd;
    final_floor2_conv_cmd = load_floor2_conv_cmd;
    final_floor3_conv_cmd = load_floor3_conv_cmd;

    % 상차 중에는 벨트4 단독 역회전/복귀 명령 없음
    final_floor1_belt4_cmd = 0;
    final_floor2_belt4_cmd = 0;
    final_floor3_belt4_cmd = 0;

% =========================
% 하차 단계
% =========================
elseif mission_phase == 1
    final_lift_cmd = unload_lift_cmd;
    final_target_z = unload_target_z;

    % 하차 준비용 전체 순환 컨베이어 명령
    final_floor1_conv_cmd = pre_floor1_conv_cmd;
    final_floor2_conv_cmd = pre_floor2_conv_cmd;
    final_floor3_conv_cmd = pre_floor3_conv_cmd;
    
    % 4번 벨트 단독 동작 중에는 전체 순환 컨베이어 정지
    if belt4_reverse_cmd == 1 || belt4_restore_cmd == 1
        final_floor1_conv_cmd = 0;
        final_floor2_conv_cmd = 0;
        final_floor3_conv_cmd = 0;
    end

    % 하차 순간 4번 벨트 단독 명령
    if target_unload_floor == 1
        if belt4_reverse_cmd == 1
            final_floor1_belt4_cmd = -1;
        elseif belt4_restore_cmd == 1
            final_floor1_belt4_cmd = 1;
        else
            final_floor1_belt4_cmd = 0;
        end

    elseif target_unload_floor == 2
        if belt4_reverse_cmd == 1
            final_floor2_belt4_cmd = -1;
        elseif belt4_restore_cmd == 1
            final_floor2_belt4_cmd = 1;
        else
            final_floor2_belt4_cmd = 0;
        end

    elseif target_unload_floor == 3
        if belt4_reverse_cmd == 1
            final_floor3_belt4_cmd = -1;
        elseif belt4_restore_cmd == 1
            final_floor3_belt4_cmd = 1;
        else
            final_floor3_belt4_cmd = 0;
        end
    end

% =========================
% 미션 완료 또는 예외
% =========================
else
    final_lift_cmd = 0;
    final_target_z = 0;
    final_pusher_cmd = 0;

    final_floor1_conv_cmd = 0;
    final_floor2_conv_cmd = 0;
    final_floor3_conv_cmd = 0;

    final_belt4_reverse_cmd = 0;
    final_belt4_restore_cmd = 0;
end

== matlab function baseline_auto_parcel_loading_process/BoxPoseFunction ==
  data: load_done input; box_yaw output
function box_yaw = BoxPoseFunction(load_done)
% BoxPoseFunction
% 택배가 플랫폼 위에 랜덤하게 놓였다고 가정하고,
% 카메라/YOLO가 인식한 초기 yaw 각도를 생성한다.
%
% box_yaw 단위: deg
% 범위: -90 deg ~ 90 deg
%
% load_done이 0 -> 1로 바뀌면 다음 택배의 yaw를 새로 생성한다.

persistent current_yaw
persistent prev_load_done

if isempty(current_yaw)
    current_yaw = -90 + 180 * rand;
    prev_load_done = 0;
end

rising_edge = (prev_load_done == 0) && (load_done == 1);

if rising_edge
    current_yaw = -90 + 180 * rand;
end

prev_load_done = load_done;

box_yaw = current_yaw;

== matlab function baseline_auto_parcel_loading_process/RotatorControlFunction ==
  data: rotator_cmd input; rotator_vel output; rotator_target_angle input; rotator_angle input; rotation_done output; rotator_home_done output
function [rotator_vel, rotation_done, rotator_home_done] = RotatorControlFunction(rotator_cmd, rotator_target_angle, rotator_angle)
% RotatorControlFunction
% rotator_cmd에 따라 회전판을 제어한다.
%
% rotator_cmd:
%   0 = 정지
%   1 = 택배 yaw 보정 목표각(rotator_target_angle)으로 회전
%   2 = 회전판 원점 0 deg로 복귀
%
% rotation_done:
%   rotator_cmd == 1일 때 목표 보정각 도달 여부
%
% rotator_home_done:
%   rotator_cmd == 2일 때 0도 복귀 완료 여부

rotator_speed = 60;   % deg/s
angle_tol = 5.0;      % deg

rotator_vel = 0;
rotation_done = 0;
rotator_home_done = 0;

if rotator_cmd == 1
    target_angle = rotator_target_angle;
    error = target_angle - rotator_angle;

    if abs(error) <= angle_tol
        rotator_vel = 0;
        rotation_done = 1;
        rotator_home_done = 0;
    else
        if error > 0
            rotator_vel = rotator_speed;
        else
            rotator_vel = -rotator_speed;
        end
        rotation_done = 0;
        rotator_home_done = 0;
    end

elseif rotator_cmd == 2
    target_angle = 0;
    error = target_angle - rotator_angle;

    if abs(error) <= angle_tol
        rotator_vel = 0;
        rotation_done = 0;
        rotator_home_done = 1;
    else
        if error > 0
            rotator_vel = rotator_speed;
        else
            rotator_vel = -rotator_speed;
        end
        rotation_done = 0;
        rotator_home_done = 0;
    end

else
    rotator_vel = 0;
    rotation_done = 0;
    rotator_home_done = 0;
end

== matlab function baseline_auto_parcel_loading_process/PusherControlFunction ==
  data: pusher_cmd input; pusher_vel output; pusher_pos input; push_done output; pusher_home_done output; push_count output
function [pusher_vel, push_done, pusher_home_done, push_count] = PusherControlFunction(pusher_cmd, pusher_pos)
% PusherControlFunction
% pusher_cmd:
%   0 = 정지
%   1 = 전진, 택배를 벨트4 방향으로 밀기
%   2 = 원점 복귀

persistent count
persistent prev_push_done

if isempty(count)
    count = 0;
    prev_push_done = 0;
end

pusher_speed = 0.05;     % m/s
push_target_pos = 0.24;  % m
pos_tol = 0.002;         % m

pusher_vel = 0;
push_done = 0;
pusher_home_done = 0;

if pusher_cmd == 1
    if pusher_pos >= push_target_pos - pos_tol
        pusher_vel = 0;
        push_done = 1;
        pusher_home_done = 0;
    else
        pusher_vel = pusher_speed;
        push_done = 0;
        pusher_home_done = 0;
    end

elseif pusher_cmd == 2
    if pusher_pos <= pos_tol
        pusher_vel = 0;
        push_done = 0;
        pusher_home_done = 1;
    else
        pusher_vel = -pusher_speed;
        push_done = 0;
        pusher_home_done = 0;
    end

else
    pusher_vel = 0;
    push_done = 0;
    pusher_home_done = 0;
end

% push_done 상승 에지 카운트
if prev_push_done == 0 && push_done == 1
    count = count + 1;
end

prev_push_done = push_done;

push_count = count;

== matlab function baseline_auto_parcel_loading_process/StopperControlFunction ==
  data: stopper_cmd input; stopper_vel output; stopper_pos input; stopper_down_done output; stopper_up_done output
function [stopper_vel, stopper_down_done, stopper_up_done] = StopperControlFunction(stopper_cmd, stopper_pos)
% StopperControlFunction
% 스토퍼 위치 모델
%
% stopper_cmd:
%   0 = 스토퍼 올림
%   1 = 스토퍼 내림
%
% stopper_pos:
%   0 = 완전히 올라간 상태
%   1 = 완전히 내려간 상태
%
% stopper_vel:
%   스토퍼 위치 변화 속도 [1/s]
%
% stopper_down_done:
%   스토퍼가 완전히 내려갔는지
%
% stopper_up_done:
%   스토퍼가 완전히 올라갔는지

stopper_speed = 2.0;   % 1/s, 0에서 1까지 약 0.5초
pos_tol = 0.01;

stopper_vel = 0;
stopper_down_done = 0;
stopper_up_done = 0;

if stopper_cmd == 1
    % 스토퍼 내림
    if stopper_pos >= 1.0 - pos_tol
        stopper_vel = 0;
        stopper_down_done = 1;
        stopper_up_done = 0;
    else
        stopper_vel = stopper_speed;
        stopper_down_done = 0;
        stopper_up_done = 0;
    end

else
    % 스토퍼 올림
    if stopper_pos <= pos_tol
        stopper_vel = 0;
        stopper_down_done = 0;
        stopper_up_done = 1;
    else
        stopper_vel = -stopper_speed;
        stopper_down_done = 0;
        stopper_up_done = 0;
    end
end

== matlab function baseline_auto_parcel_loading_process/StopperCommandFunction ==
  data: mission_phase input; stopper_cmd_final output; loading_enable input
function stopper_cmd_final = StopperCommandFunction(mission_phase, loading_enable)
% StopperCommandFunction
% 스토퍼는 택배 1개마다 올렸다 내리는 것이 아니라,
% 상차 phase 동안 계속 내려와 있고,
% 상차가 끝난 뒤에만 올라간다.
%
% mission_phase:
%   0 = 상차 단계
%   1 = 하차 단계
%   2 = 미션 완료
%
% loading_enable:
%   1 = 상차 허용
%   0 = 상차 종료

if mission_phase == 0 && loading_enable == 1
    stopper_cmd_final = 1;   % 상차 중: 스토퍼 내림 유지
else
    stopper_cmd_final = 0;   % 상차 종료/하차/완료: 스토퍼 올림
end

== matlab function baseline_auto_parcel_loading_process/PackageSlotVisualizer ==
  data: floor1_queue input size=[50 1]; floor1_slot_id output size=[50 1]; floor2_queue input size=[50 1]; floor3_queue input size=[50 1]; sensor_count_f1 input size=[1 1]; floor2_slot_id output size=[50 1]; floor3_slot_id output size=[50 1]; sensor_count_f2 input size=[1 1]; sensor_count_f3 input size=[1 1]
function [floor1_slot_id, floor2_slot_id, floor3_slot_id] = ...
    PackageSlotVisualizer(floor1_queue, floor2_queue, floor3_queue, ...
                          sensor_count_f1, sensor_count_f2, sensor_count_f3)
% PackageSlotVisualizer
%
% 목적:
% - FloorStorageUpdate에 저장된 각 층 queue를 기반으로,
%   3D 표시용 slot_id 배열을 만든다.
%
% 핵심:
% - 실제 queue 자체를 회전시키지 않는다.
% - 하차 준비 중 컨베이어가 회전한 만큼만 시각화용 slot_id를 회전한다.
% - 각 층은 독립적으로 회전한다.
%
% 입력:
% floor1_queue      [50x1]
% floor2_queue      [50x1]
% floor3_queue      [50x1]
% sensor_count_f1   [1x1]
% sensor_count_f2   [1x1]
% sensor_count_f3   [1x1]
%
% 출력:
% floor1_slot_id    [50x1]
% floor2_slot_id    [50x1]
% floor3_slot_id    [50x1]
%
% 예:
% floor2_queue = [1 2 3 4 5 6 0 ...]
% sensor_count_f2 = 3
% floor2_slot_id = [4 5 6 1 2 3 0 ...]

QUEUE_MAX = 50;

floor1_slot_id = zeros(QUEUE_MAX, 1);
floor2_slot_id = zeros(QUEUE_MAX, 1);
floor3_slot_id = zeros(QUEUE_MAX, 1);

floor1_slot_id = rotateQueueForDisplay(floor1_queue, sensor_count_f1, QUEUE_MAX);
floor2_slot_id = rotateQueueForDisplay(floor2_queue, sensor_count_f2, QUEUE_MAX);
floor3_slot_id = rotateQueueForDisplay(floor3_queue, sensor_count_f3, QUEUE_MAX);

end


function slot_id = rotateQueueForDisplay(queue, sensor_count, queue_max)
% rotateQueueForDisplay
%
% queue 안의 유효 package_id만 추출한 뒤,
% sensor_count만큼 앞에서 뒤로 회전시킨 표시용 배열을 만든다.
%
% queue 자체는 바꾸지 않는다.

slot_id = zeros(queue_max, 1);

% =========================
% 유효 package 추출
% =========================
valid = zeros(queue_max, 1);
n = 0;

for i = 1:queue_max
    if queue(i) > 0
        n = n + 1;
        valid(n) = queue(i);
    end
end

if n <= 0
    return;
end

% =========================
% sensor_count 정리
% =========================
shift = int32(sensor_count);

if shift < 0
    shift = int32(0);
end

% n개 기준으로 회전
% 예: n=6, shift=6이면 원래 순서로 복귀
while shift >= n
    shift = shift - n;
end

% =========================
% 회전 표시
% =========================
% sensor_count = 0:
%   [1 2 3 4 5 6]
%
% sensor_count = 1:
%   [2 3 4 5 6 1]
%
% sensor_count = 3:
%   [4 5 6 1 2 3]
for out_idx = 1:n
    src_idx = out_idx + shift;

    while src_idx > n
        src_idx = src_idx - n;
    end

    slot_id(out_idx) = valid(src_idx);
end

end

== matlab function baseline_auto_parcel_loading_process/PackageSlotToXYZFunction ==
  data: floor1_slot_id input size=[50 1]; floor2_slot_id input size=[50 1]; floor3_slot_id input size=[50 1]; target_id_f1 input size=[1 1]; target_on_belt4_f1 input size=[1 1]; target_id_f2 input size=[1 1]; floor1_visible output size=[50 1]; floor1_color_flag output size=[50 1]; floor2_visible output size=[50 1]; floor2_color_flag output size=[50 1]; floor3_visible output size=[50 1]; floor3_color_flag output size=[50 1]; target_on_belt4_f2 input size=[1 1]; target_id_f3 input size=[1 1]; target_on_belt4_f3 input size=[1 1]
function [floor1_visible, floor1_color_flag, ...
          floor2_visible, floor2_color_flag, ...
          floor3_visible, floor3_color_flag] = ...
          PackageSlotToXYZFunction(floor1_slot_id, floor2_slot_id, floor3_slot_id, ...
                                   target_id_f1, target_on_belt4_f1, ...
                                   target_id_f2, target_on_belt4_f2, ...
                                   target_id_f3, target_on_belt4_f3)
% PackageSlotToXYZFunction
%
% 목적:
% - PackageSlotVisualizer에서 만든 floorN_slot_id를 받아
%   각 층의 표시 여부 visible과 색상 flag를 만든다.
%
% 입력:
% floor1_slot_id      [50x1]
% floor2_slot_id      [50x1]
% floor3_slot_id      [50x1]
%
% target_id_f1        [1x1]
% target_on_belt4_f1  [1x1]
% target_id_f2        [1x1]
% target_on_belt4_f2  [1x1]
% target_id_f3        [1x1]
% target_on_belt4_f3  [1x1]
%
% 출력:
% floorN_visible      [50x1]
% floorN_color_flag   [50x1]
%
% 규칙:
% - slot_id > 0 이면 visible = 1
% - 해당 slot_id가 그 층의 target_id_fN이고 target_on_belt4_fN = 1이면 color_flag = 1
% - 그 외에는 color_flag = 0
%
% 주의:
% - floorN_highlight 같은 [50x1] 배열 입력을 더 이상 사용하지 않는다.
% - target_on_belt4_fN은 scalar이므로 floorN_highlight(i)처럼 인덱싱하면 안 된다.

QUEUE_MAX = 50;

floor1_visible = zeros(QUEUE_MAX, 1);
floor2_visible = zeros(QUEUE_MAX, 1);
floor3_visible = zeros(QUEUE_MAX, 1);

floor1_color_flag = zeros(QUEUE_MAX, 1);
floor2_color_flag = zeros(QUEUE_MAX, 1);
floor3_color_flag = zeros(QUEUE_MAX, 1);

% =========================
% 1층
% =========================
for i = 1:QUEUE_MAX
    pkg_id = floor1_slot_id(i);

    if pkg_id > 0
        floor1_visible(i) = 1;
    else
        floor1_visible(i) = 0;
    end

    if target_on_belt4_f1 > 0.5 && target_id_f1 > 0 && pkg_id == target_id_f1
        floor1_color_flag(i) = 1;
    else
        floor1_color_flag(i) = 0;
    end
end

% =========================
% 2층
% =========================
for i = 1:QUEUE_MAX
    pkg_id = floor2_slot_id(i);

    if pkg_id > 0
        floor2_visible(i) = 1;
    else
        floor2_visible(i) = 0;
    end

    if target_on_belt4_f2 > 0.5 && target_id_f2 > 0 && pkg_id == target_id_f2
        floor2_color_flag(i) = 1;
    else
        floor2_color_flag(i) = 0;
    end
end

% =========================
% 3층
% =========================
for i = 1:QUEUE_MAX
    pkg_id = floor3_slot_id(i);

    if pkg_id > 0
        floor3_visible(i) = 1;
    else
        floor3_visible(i) = 0;
    end

    if target_on_belt4_f3 > 0.5 && target_id_f3 > 0 && pkg_id == target_id_f3
        floor3_color_flag(i) = 1;
    else
        floor3_color_flag(i) = 0;
    end
end

end

== matlab function baseline_auto_parcel_loading_process/VisualizationPacketFunction ==
  data: mission_phase input; vis_platform_z output; state_id input; unload_state_id input; platform_z input; rotator_angle input; pusher_pos input; stopper_pos input; final_lift_cmd input; final_floor1_conv_cmd input; final_floor2_conv_cmd input; final_floor3_conv_cmd input; final_floor1_belt4_cmd input; final_floor2_belt4_cmd input; final_floor3_belt4_cmd input; floor1_x input; floor1_y input; floor1_z input; floor1_yaw input; floor1_visible input; floor1_color_flag input; floor2_x input; floor2_y input; floor2_z input; floor2_yaw input; floor2_visible input; floor2_color_flag input; floor3_x input; floor3_y input; floor3_z input; floor3_yaw input; floor3_visible input; floor3_color_flag input; vis_rotator_angle output; vis_pusher_pos output; vis_stopper_pos output; vis_mission_phase output; vis_load_state output; vis_unload_state output; vis_lift_cmd output; vis_floor1_conv_cmd output; vis_floor2_conv_cmd output; vis_floor3_conv_cmd output; vis_floor1_belt4_cmd output; vis_floor2_belt4_cmd output; vis_floor3_belt4_cmd output; vis_floor1_x output; vis_floor1_y output; vis_floor1_z output; vis_floor1_yaw output; vis_floor1_visible output; vis_floor1_color_flag output; vis_floor2_x output; vis_floor2_y output; vis_floor2_z output; vis_floor2_yaw output; vis_floor2_visible output; vis_floor2_color_flag output; vis_floor3_x output; vis_floor3_y output; vis_floor3_z output; vis_floor3_yaw output; vis_floor3_visible output; vis_floor3_color_flag output
function [vis_platform_z, vis_rotator_angle, vis_pusher_pos, vis_stopper_pos, ...
    vis_mission_phase, vis_load_state, vis_unload_state, ...
    vis_lift_cmd, ...
    vis_floor1_conv_cmd, vis_floor2_conv_cmd, vis_floor3_conv_cmd, ...
    vis_floor1_belt4_cmd, vis_floor2_belt4_cmd, vis_floor3_belt4_cmd, ...
    vis_floor1_x, vis_floor1_y, vis_floor1_z, vis_floor1_yaw, vis_floor1_visible, vis_floor1_color_flag, ...
    vis_floor2_x, vis_floor2_y, vis_floor2_z, vis_floor2_yaw, vis_floor2_visible, vis_floor2_color_flag, ...
    vis_floor3_x, vis_floor3_y, vis_floor3_z, vis_floor3_yaw, vis_floor3_visible, vis_floor3_color_flag] = ...
    VisualizationPacketFunction(mission_phase, state_id, unload_state_id, ...
    platform_z, rotator_angle, pusher_pos, stopper_pos, ...
    final_lift_cmd, ...
    final_floor1_conv_cmd, final_floor2_conv_cmd, final_floor3_conv_cmd, ...
    final_floor1_belt4_cmd, final_floor2_belt4_cmd, final_floor3_belt4_cmd, ...
    floor1_x, floor1_y, floor1_z, floor1_yaw, floor1_visible, floor1_color_flag, ...
    floor2_x, floor2_y, floor2_z, floor2_yaw, floor2_visible, floor2_color_flag, ...
    floor3_x, floor3_y, floor3_z, floor3_yaw, floor3_visible, floor3_color_flag)
% VisualizationPacketFunction
% 3D 시각화 연동용 최종 출력 패킷 정리 함수
%
% 현재 단계에서는 입력 신호를 3D 시각화용 이름으로 정리해서 그대로 출력한다.
% 나중에 Unity UDP/TCP 송신, Simulink 3D Animation, App Designer 등으로 연결할 수 있다.

% =========================
% Actuator visualization
% =========================
vis_platform_z = platform_z;
vis_rotator_angle = rotator_angle;
vis_pusher_pos = pusher_pos;
vis_stopper_pos = stopper_pos;

% =========================
% Mission/state visualization
% =========================
vis_mission_phase = mission_phase;
vis_load_state = state_id;
vis_unload_state = unload_state_id;

% =========================
% Final command visualization
% =========================
vis_lift_cmd = final_lift_cmd;

vis_floor1_conv_cmd = final_floor1_conv_cmd;
vis_floor2_conv_cmd = final_floor2_conv_cmd;
vis_floor3_conv_cmd = final_floor3_conv_cmd;

vis_floor1_belt4_cmd = final_floor1_belt4_cmd;
vis_floor2_belt4_cmd = final_floor2_belt4_cmd;
vis_floor3_belt4_cmd = final_floor3_belt4_cmd;

% =========================
% Package visualization
% =========================
vis_floor1_x = floor1_x;
vis_floor1_y = floor1_y;
vis_floor1_z = floor1_z;
vis_floor1_yaw = floor1_yaw;
vis_floor1_visible = floor1_visible;
vis_floor1_color_flag = floor1_color_flag;

vis_floor2_x = floor2_x;
vis_floor2_y = floor2_y;
vis_floor2_z = floor2_z;
vis_floor2_yaw = floor2_yaw;
vis_floor2_visible = floor2_visible;
vis_floor2_color_flag = floor2_color_flag;

vis_floor3_x = floor3_x;
vis_floor3_y = floor3_y;
vis_floor3_z = floor3_z;
vis_floor3_yaw = floor3_yaw;
vis_floor3_visible = floor3_visible;
vis_floor3_color_flag = floor3_color_flag;
